simulink library "dragTurbineNew_ul"  (R2020a)
settings: Solver=VariableStepAuto  StartTime=0.0  StopTime=10.0  RelTol=1e-3
undefined symbols (not defined in the file): vhcl
libraries: dragTurbineVaryCpCt_ul x2
settings Model: Creator=Ayaz  LastModifiedBy=mr-jo
settings DataIOCC: ReturnWorkspaceOutputs=off
settings DebuggingCC: ArithmeticOperatorsInVariantConditions=warning
settings SFSimCC: CustomCodeUndefinedFunction=UseInterfaceOnly

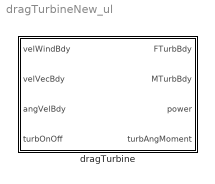
== system dragTurbineNew_ul ==
  dragTurbine : Subsystem  TreatAsAtomicUnit=on

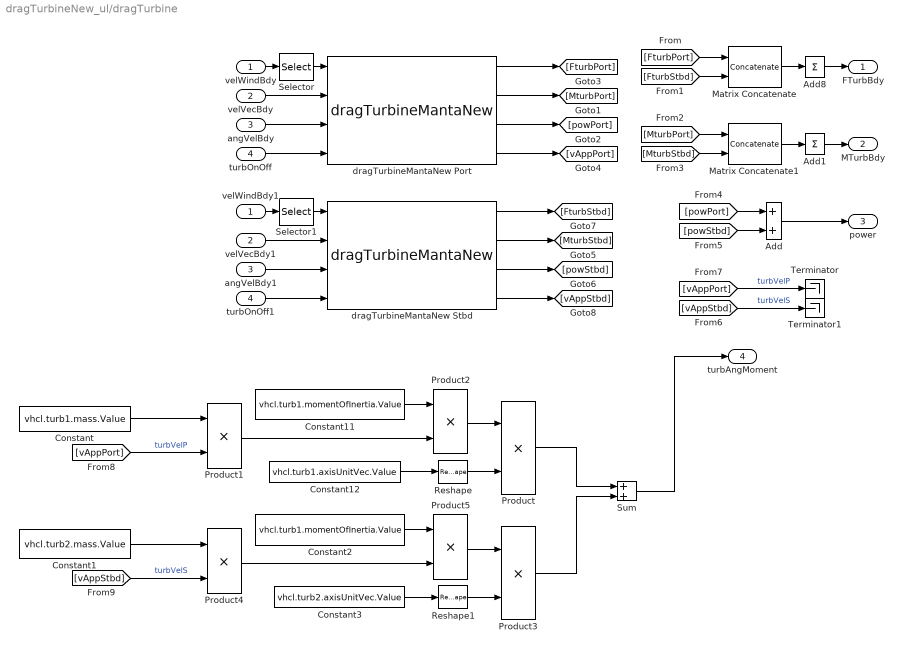
== system dragTurbineNew_ul/dragTurbine ==
  velWindBdy : Inport
  velVecBdy : Inport  Port=2
  angVelBdy : Inport  Port=3
  turbOnOff : Inport  Port=4
  Add : Sum
  Add1 : Sum  Inputs=1  CollapseMode=Specified dimension  CollapseDim=2
  Add8 : Sum  Inputs=1  CollapseMode=Specified dimension  CollapseDim=2
  Constant : Constant  Value=vhcl.turb1.mass.Value
  Constant1 : Constant  Value=vhcl.turb2.mass.Value
  Constant11 : Constant  Value=vhcl.turb1.momentOfInertia.Value
  Constant12 : Constant  Value=vhcl.turb1.axisUnitVec.Value
  Constant2 : Constant  Value=vhcl.turb1.momentOfInertia.Value
  Constant3 : Constant  Value=vhcl.turb2.axisUnitVec.Value
  Matrix Concatenate : Concatenate  Mode=Multidimensional array  ConcatenateDimension=2
  Matrix Concatenate1 : Concatenate  Mode=Multidimensional array  ConcatenateDimension=2
  Product{,1..5} (6 alike) : Product
  Reshape : Reshape  OutputDimensionality=Column vector (2-D)
  Reshape1 : Reshape  OutputDimensionality=Column vector (2-D)
  Selector : Selector  NumberOfDimensions=2  InputPortWidth=3  IndexOptions=Index vector (dialog),Index vector (dialog)  Indices=[1 2 3],1  OutputSizes=1,1
  Selector1 : Selector  NumberOfDimensions=2  InputPortWidth=3  IndexOptions=Index vector (dialog),Index vector (dialog)  Indices=[1 2 3],2  OutputSizes=1,1
  Sum : Sum
  Terminator : Terminator
  Terminator1 : Terminator
  angVelBdy1 : InportShadow  Port=3
  dragTurbineMantaNew Port : dragTurbineVaryCpCt_ul/dragTurbineMantaNew  rho_fluid=rho  turb_struct=vcl.turb1
  dragTurbineMantaNew Stbd : dragTurbineVaryCpCt_ul/dragTurbineMantaNew  rho_fluid=rho  turb_struct=vcl.turb2
  turbOnOff1 : InportShadow  Port=4
  velVecBdy1 : InportShadow  Port=2
  velWindBdy1 : InportShadow
  FTurbBdy : Outport  PortDimensions=[3,1]  VectorParamsAs1DForOutWhenUnconnected=off
  MTurbBdy : Outport  Port=2  PortDimensions=[3,1]  VectorParamsAs1DForOutWhenUnconnected=off
  power : Outport  Port=3  PortDimensions=[1,1]  VectorParamsAs1DForOutWhenUnconnected=off
  turbAngMoment : Outport  Port=4  PortDimensions=[3,1]  VectorParamsAs1DForOutWhenUnconnected=off
  wires:
  velVecBdy/1 -> dragTurbineMantaNew Port/2
  angVelBdy/1 -> dragTurbineMantaNew Port/3
  turbOnOff/1 -> dragTurbineMantaNew Port/4
  velVecBdy1/1 -> dragTurbineMantaNew Stbd/2
  angVelBdy1/1 -> dragTurbineMantaNew Stbd/3
  turbOnOff1/1 -> dragTurbineMantaNew Stbd/4
  dragTurbineMantaNew Port/1 -> [FturbPort]
  dragTurbineMantaNew Port/4 -> [vAppPort]
  dragTurbineMantaNew Port/3 -> [powPort]
  dragTurbineMantaNew Port/2 -> [MturbPort]
  dragTurbineMantaNew Stbd/4 -> [vAppStbd]
  dragTurbineMantaNew Stbd/3 -> [powStbd]
  dragTurbineMantaNew Stbd/2 -> [MturbStbd]
  dragTurbineMantaNew Stbd/1 -> [FturbStbd]
  Matrix Concatenate/1 -> Add8/1
  Matrix Concatenate1/1 -> Add1/1
  [FturbPort] -> Matrix Concatenate/1
  [FturbStbd] -> Matrix Concatenate/2
  [MturbPort] -> Matrix Concatenate1/1
  [MturbStbd] -> Matrix Concatenate1/2
  [vAppPort] -> Terminator/1  "turbVelP"
  [vAppStbd] -> Terminator1/1  "turbVelS"
  velWindBdy/1 -> Selector/1
  Selector/1 -> dragTurbineMantaNew Port/1
  Selector1/1 -> dragTurbineMantaNew Stbd/1
  velWindBdy1/1 -> Selector1/1
  Add8/1 -> FTurbBdy/1
  Add1/1 -> MTurbBdy/1
  [powPort] -> Add/1
  [powStbd] -> Add/2
  Add/1 -> power/1
  Product1/1 -> Product2/2
  Constant11/1 -> Product2/1
  Product2/1 -> Product/1
  Reshape/1 -> Product/2
  Constant12/1 -> Reshape/1
  [vAppPort] -> Product1/2  "turbVelP"
  Constant/1 -> Product1/1
  Constant1/1 -> Product4/1
  Constant3/1 -> Reshape1/1
  Product5/1 -> Product3/1
  Constant2/1 -> Product5/1
  Reshape1/1 -> Product3/2
  Product4/1 -> Product5/2
  [vAppStbd] -> Product4/2  "turbVelS"
  Product/1 -> Sum/1
  Product3/1 -> Sum/2
  Sum/1 -> turbAngMoment/1
